simulink model "PlanarRobot5link_changedconstraint"  (R2022b)
settings: Solver=VariableStepAuto  StartTime=0.0  StopTime=100  RelTol=1e-3
values from neighbouring files (symbols this model uses):
  I = [1; 1; 1; 0.5; 0.5]*0.2    [RobDyn4link.m]
  l = [1; 1; 1; 1; 2]*0.2    [RobDyn4link.m]
  lc = l./2    [RobDyn4link.m]
  m = [1; 1; 1; 0.3; 0.3]*1    [RobDyn4link.m]
  q0 = [pi/2; -pi/4; -1*pi/6;-pi/12;0;]    [RobDyn4link.m]
  theta_max = [0.915*pi; 0.915*pi; 0.915*pi; 0.915*pi; 0.915*pi;]    [RobDyn4link.m]
  theta_min = [-0.915*pi; -0.915*pi; -0.915*pi; -0.915*pi; -0.915*pi;]    [RobDyn4link.m]
libraries: slpidlib x2
(part 1 of 3)
settings Model: Creator=yu  LastModifiedBy=ge89moy

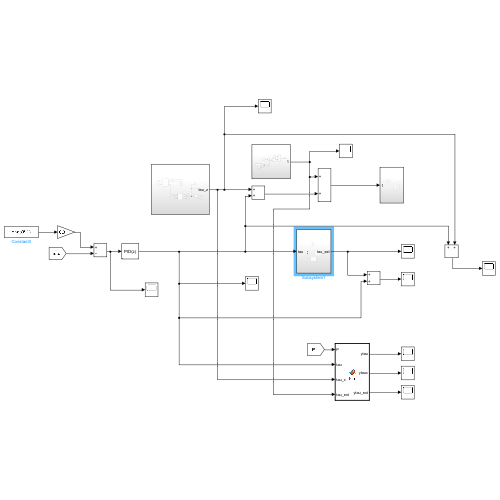
[thumbnail: Simulink's stored preview of the top-level diagram]
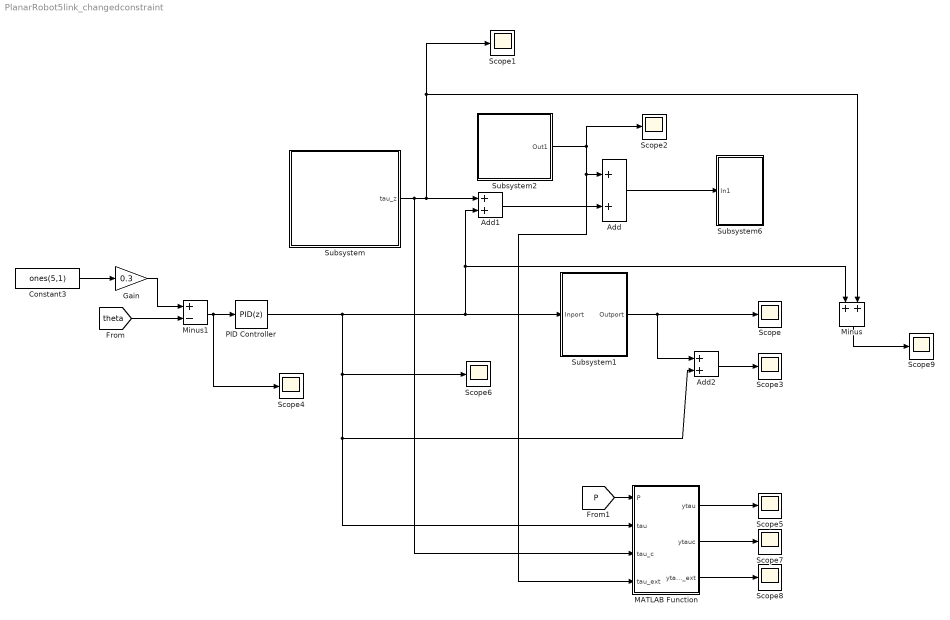
== system PlanarRobot5link_changedconstraint ==
  Add : Sum
  Add1 : Sum
  Add2 : Sum
  Constant3 : Constant  Value=ones(5,1)
  Gain : Gain  Gain=0.3
  MATLAB Function : MATLAB Function  TreatAsAtomicUnit=on
  Minus : Sum
  Minus1 : Sum  Inputs=+-
  PID Controller : slpidlib/PID Controller  Controller=PID  Form=Parallel  TimeDomain=Discrete-time  UseExternalTs=off  SampleTime=1e-3  IntegratorMethod=Forward Euler  FilterMethod=Forward Euler  ControllerParametersSource=internal  P=100  I=0  UseKiTs=off  D=50  N=100  UseFilter=on  TunerSelectOption=Transfer Function Based (PID Tuner App)  InitialConditionSource=internal  InitialConditionForIntegrator=0  InitialConditionForFilter=0  DifferentiatorICPrevScaledInput=0  ExternalReset=none  TrackingMode=off  Kt=1  LimitOutput=off  SatLimitsSource=internal  UpperSaturationLimit=inf  LowerSaturationLimit=-inf  LinearizeAsGain=on  AntiWindupMode=none  Kb=1  LimitIntegrator=off  UpperIntegratorSaturationLimit=inf  LowerIntegratorSaturationLimit=-inf  POutMin=[]  POutMax=[]  IOutMin=[]  IOutMax=[]  DOutMin=[]  DOutMax=[]  NOutMin=[]  NOutMax=[]  SumOutMin=[]  SumOutMax=[]  SaturationOutMin=[]  SaturationOutMax=[]  PParamMin=[]  PParamMax=[]  IParamMin=[]  IParamMax=[]  DParamMin=[]  DParamMax=[]  NParamMin=[]  NParamMax=[]  KbParamMin=[]  KbParamMax=[]  KtParamMin=[]  KtParamMax=[]  KbOutMin=[]  KbOutMax=[]  KtOutMin=[]  KtOutMax=[]  IntegratorOutMin=[]  IntegratorOutMax=[]  FilterOutMin=[]  FilterOutMax=[]  SumI1OutMin=[]  SumI1OutMax=[]  SumI2OutMin=[]  SumI2OutMax=[]  SumI3OutMin=[]  SumI3OutMax=[]  SumI4OutMin=[]  SumI4OutMax=[]  SumDOutMin=[]  SumDOutMax=[]  DifferentiatorOutMin=[]  DifferentiatorOutMax=[]  FilterDiffOutCoefMin=[]  FilterDiffOutCoefMax=[]  ReciprocalOutMin=[]  ReciprocalOutMax=[]  SumDenOutMin=[]  SumDenOutMax=[]  SumNumOutMin=[]  SumNumOutMax=[]  DivideOutMin=[]  DivideOutMax=[]  UdiffTsProdOutMin=[]  UdiffTsProdOutMax=[]  NTsProdOutMin=[]  NTsProdOutMax=[]  UintegralTsProdOutMin=[]  UintegralTsProdOutMax=[]  UngainTsProdOutMin=[]  UngainTsProdOutMax=[]  ClampingZeroOutDataTypeStr=Inherit: Inherit via back propagation  ClampingZeroOutMin=[]  ClampingZeroOutMax=[]  FilterDenConstantOutDataTypeStr=Inherit: Inherit via back propagation  FilterDenConstantOutMin=[]  FilterDenConstantOutMax=[]  PCopyOutDataTypeStr=Inherit: Inherit via back propagation  PCopyOutMin=[]  PCopyOutMax=[]  NCopyOutDataTypeStr=Inherit: Inherit via back propagation  NCopyOutMin=[]  NCopyOutMax=[]  IntegratorContinuousStateAttributes=''  IntegratorStateMustResolveToSignalObject=off  IntegratorRTWStateStorageClass=Auto  FilterContinuousStateAttributes=''  FilterStateMustResolveToSignalObject=off  FilterRTWStateStorageClass=Auto  ParallelPVariant=InternalParameters  IdealPVariant=Disabled  IVariant=InternalParameters  DVariant=InternalParameters  IntegratorVariant=Discrete  SatVariant=Disabled  AWVariant=Passthrough  PCopyVariant=Disabled  TRVariant=Disabled  FdbkBlocksVariant=Forward  IdealPFdbkVariant=Disabled  SatFdbkVariant=Disabled  DerivativeFilterVariant=ForwardEulerFilter  NVariant=InternalParameters  NCopyVariant=Disabled  FilterICVariant=InternalICsFilter  IntegratorICVariant=InternalICs  ExternalResetVariant=Disabled  TRSumVariant=Passthrough  SumFdbkVariant=Disabled  SumVariant=Sum_PID  TsampFilterVariant=InternalTs  TsampNgainVariant=Passthrough  TsampIntegralVariant=Passthrough  ExternalSaturationOutDataTypeStr=Inherit: Same as second input
  Scope{,1..9} (10 alike) : Scope
  Subsystem : Subsystem
  Subsystem1 : Subsystem
  Subsystem2 : Subsystem
  Subsystem6 : Subsystem
  wires:
  Minus1/1 -> Scope4/1, PID Controller/1
  Add1/1 -> Add/2
  Constant3/1 -> Gain/1
  [theta] -> Minus1/2
  Add/1 -> Subsystem6/1(In1)
  Gain/1 -> Minus1/1
  Subsystem/1(tau_z) -> Add1/1, Scope1/1, Minus/2, MATLAB Function/3(tau_c)
  PID Controller/1 -> Add1/2, Minus/1, Subsystem1/1(Inport), Add2/2, MATLAB Function/2(tau), Scope6/1
  Subsystem1/1(Outport) -> Add2/1, Scope/1
  Add2/1 -> Scope3/1
  [P] -> MATLAB Function/1(P)
  MATLAB Function/1(ytau) -> Scope5/1
  MATLAB Function/2(ytauc) -> Scope7/1
  MATLAB Function/3(ytau_ext) -> Scope8/1
  Subsystem2/1(Out1) -> Add/1, MATLAB Function/4(tau_ext), Scope2/1
  Minus/1 -> Scope9/1

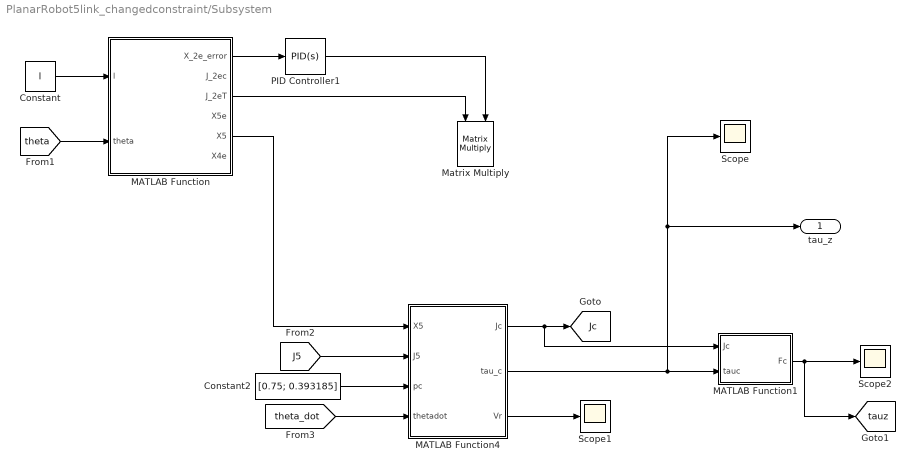
== system PlanarRobot5link_changedconstraint/Subsystem ==
  Constant : Constant  Value=l
  Constant2 : Constant  Value=[0.75; 0.393185]
  MATLAB Function : MATLAB Function  TreatAsAtomicUnit=on
  MATLAB Function1 : MATLAB Function  TreatAsAtomicUnit=on
  MATLAB Function4 : MATLAB Function  TreatAsAtomicUnit=on
  Matrix Multiply : Product  Multiplication=Matrix(*)
  PID Controller1 : slpidlib/PID Controller  Controller=PID  Form=Parallel  TimeDomain=Continuous-time  UseExternalTs=off  SampleTime=-1  IntegratorMethod=Forward Euler  FilterMethod=Forward Euler  ControllerParametersSource=internal  P=1e5  I=0  UseKiTs=off  D=1e3  N=100  UseFilter=on  TunerSelectOption=Transfer Function Based (PID Tuner App)  InitialConditionSource=internal  InitialConditionForIntegrator=0  InitialConditionForFilter=0  DifferentiatorICPrevScaledInput=0  ExternalReset=none  TrackingMode=off  Kt=1  LimitOutput=off  SatLimitsSource=internal  UpperSaturationLimit=inf  LowerSaturationLimit=-inf  LinearizeAsGain=on  AntiWindupMode=none  Kb=1  LimitIntegrator=off  UpperIntegratorSaturationLimit=inf  LowerIntegratorSaturationLimit=-inf  POutMin=[]  POutMax=[]  IOutMin=[]  IOutMax=[]  DOutMin=[]  DOutMax=[]  NOutMin=[]  NOutMax=[]  SumOutMin=[]  SumOutMax=[]  SaturationOutMin=[]  SaturationOutMax=[]  PParamMin=[]  PParamMax=[]  IParamMin=[]  IParamMax=[]  DParamMin=[]  DParamMax=[]  NParamMin=[]  NParamMax=[]  KbParamMin=[]  KbParamMax=[]  KtParamMin=[]  KtParamMax=[]  KbOutMin=[]  KbOutMax=[]  KtOutMin=[]  KtOutMax=[]  IntegratorOutMin=[]  IntegratorOutMax=[]  FilterOutMin=[]  FilterOutMax=[]  SumI1OutMin=[]  SumI1OutMax=[]  SumI2OutMin=[]  SumI2OutMax=[]  SumI3OutMin=[]  SumI3OutMax=[]  SumI4OutMin=[]  SumI4OutMax=[]  SumDOutMin=[]  SumDOutMax=[]  DifferentiatorOutMin=[]  DifferentiatorOutMax=[]  FilterDiffOutCoefMin=[]  FilterDiffOutCoefMax=[]  ReciprocalOutMin=[]  ReciprocalOutMax=[]  SumDenOutMin=[]  SumDenOutMax=[]  SumNumOutMin=[]  SumNumOutMax=[]  DivideOutMin=[]  DivideOutMax=[]  UdiffTsProdOutMin=[]  UdiffTsProdOutMax=[]  NTsProdOutMin=[]  NTsProdOutMax=[]  UintegralTsProdOutMin=[]  UintegralTsProdOutMax=[]  UngainTsProdOutMin=[]  UngainTsProdOutMax=[]  ClampingZeroOutDataTypeStr=Inherit: Inherit via back propagation  ClampingZeroOutMin=[]  ClampingZeroOutMax=[]  FilterDenConstantOutDataTypeStr=Inherit: Inherit via back propagation  FilterDenConstantOutMin=[]  FilterDenConstantOutMax=[]  PCopyOutDataTypeStr=Inherit: Inherit via back propagation  PCopyOutMin=[]  PCopyOutMax=[]  NCopyOutDataTypeStr=Inherit: Inherit via back propagation  NCopyOutMin=[]  NCopyOutMax=[]  IntegratorContinuousStateAttributes=''  IntegratorStateMustResolveToSignalObject=off  IntegratorRTWStateStorageClass=Auto  FilterContinuousStateAttributes=''  FilterStateMustResolveToSignalObject=off  FilterRTWStateStorageClass=Auto  ParallelPVariant=InternalParameters  IdealPVariant=Disabled  IVariant=InternalParameters  DVariant=InternalParameters  IntegratorVariant=Continuous  SatVariant=Disabled  AWVariant=Passthrough  PCopyVariant=Disabled  TRVariant=Disabled  FdbkBlocksVariant=Forward  IdealPFdbkVariant=Disabled  SatFdbkVariant=Disabled  DerivativeFilterVariant=ContFilter  NVariant=InternalParameters  NCopyVariant=Disabled  FilterICVariant=InternalICsFilter  IntegratorICVariant=InternalICs  ExternalResetVariant=Disabled  TRSumVariant=Passthrough  SumFdbkVariant=Disabled  SumVariant=Sum_PID  TsampFilterVariant=InternalTs  TsampNgainVariant=Passthrough  TsampIntegralVariant=Passthrough  ExternalSaturationOutDataTypeStr=Inherit: Same as second input
  Scope : Scope
  Scope1 : Scope
  Scope2 : Scope
  tau_z : Outport
  tag scope: Jc=global, tauz=global
  wires:
  MATLAB Function4/2(tau_c) -> MATLAB Function1/2(tauc), Scope/1, tau_z/1
  PID Controller1/1 -> Matrix Multiply/2
  Constant/1 -> MATLAB Function/1(l)
  [theta] -> MATLAB Function/2(theta)
  MATLAB Function/3(J_2eT) -> Matrix Multiply/1
  MATLAB Function/1(X_2e_error) -> PID Controller1/1
  MATLAB Function/5(X5) -> MATLAB Function4/1(X5)
  Constant2/1 -> MATLAB Function4/3(pc)
  [J5] -> MATLAB Function4/2(J5)
  [theta_dot] -> MATLAB Function4/4(thetadot)
  MATLAB Function4/1(Jc) -> MATLAB Function1/1(Jc), [Jc]
  MATLAB Function4/3(Vr) -> Scope1/1
  MATLAB Function1/1(Fc) -> [tauz], Scope2/1

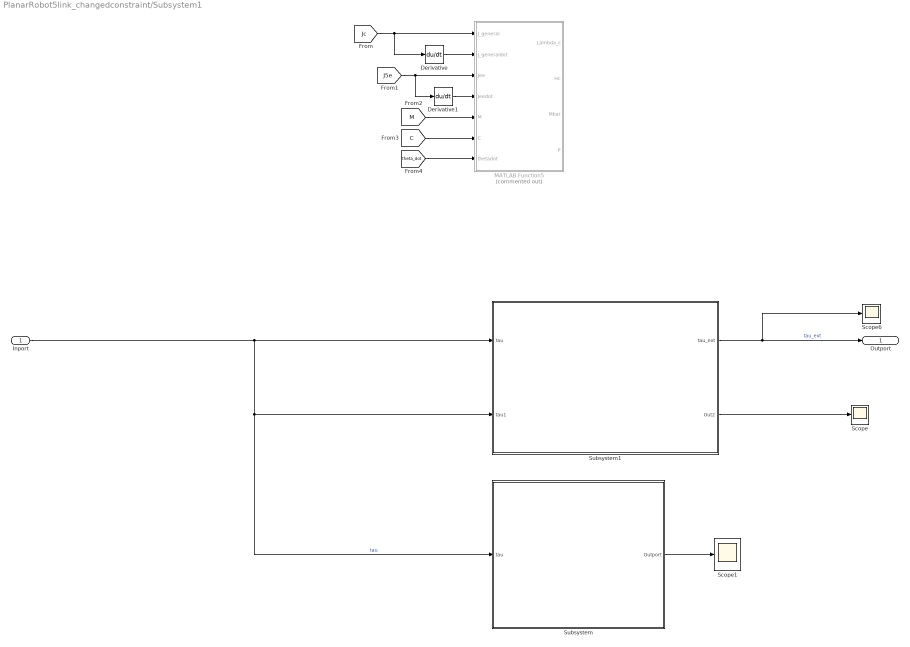
== system PlanarRobot5link_changedconstraint/Subsystem1 ==
  Inport : Inport
  Derivative : Derivative
  Derivative1 : Derivative
  MATLAB Function5 : MATLAB Function  Commented=on  TreatAsAtomicUnit=on
  Scope : Scope
  Scope1 : Scope
  Scope6 : Scope
  Subsystem : Subsystem
  Subsystem1 : Subsystem
  Outport : Outport
  wires:
  Inport/1 -> Subsystem/1(tau), Subsystem1/2(tau1), Subsystem1/1(tau)  "tau"
  Subsystem/1(Outport) -> Scope1/1
  Subsystem1/1(tau_ext) -> Outport/1, Scope6/1  "tau_ext"
  Subsystem1/2(Out2) -> Scope/1
  [Jc] -> Derivative/1, MATLAB Function5/1(J_general)
  Derivative/1 -> MATLAB Function5/2(J_generaldot)
  [J5e] -> Derivative1/1, MATLAB Function5/3(Jee)
  Derivative1/1 -> MATLAB Function5/4(Jeedot)
  [M] -> MATLAB Function5/5(M)
  [C] -> MATLAB Function5/6(C)
  [theta_dot] -> MATLAB Function5/7(thetadot)

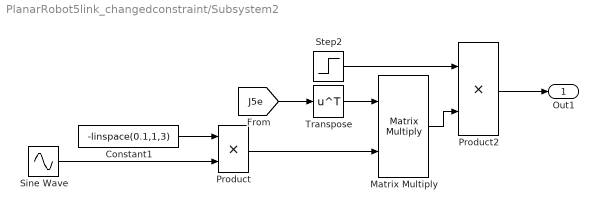
== system PlanarRobot5link_changedconstraint/Subsystem2 ==
  Constant1 : Constant  Value=-linspace(0.1,1,3)
  Matrix Multiply : Product  Multiplication=Matrix(*)
  Product : Product
  Product2 : Product
  Sine Wave : Sin  Frequency=0.1  SampleTime=0
  Step2 : Step  Time=15  After=5  SampleTime=0
  Transpose : Math  Operator=transpose
  Out1 : Outport
  wires:
  [J5e] -> Transpose/1
  Transpose/1 -> Matrix Multiply/1
  Product/1 -> Matrix Multiply/2
  Matrix Multiply/1 -> Product2/2
  Product2/1 -> Out1/1
  Step2/1 -> Product2/1
  Constant1/1 -> Product/1
  Sine Wave/1 -> Product/2

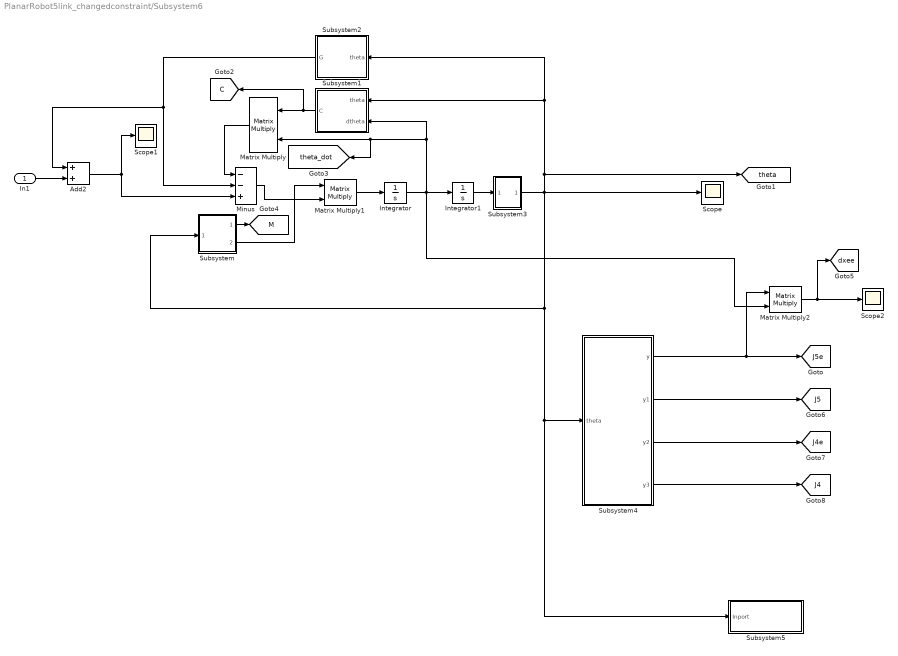
== system PlanarRobot5link_changedconstraint/Subsystem6 ==
  In1 : Inport
  Add2 : Sum
  Integrator : Integrator
  Integrator1 : Integrator  InitialCondition=q0
  Matrix Multiply : Product  Multiplication=Matrix(*)
  Matrix Multiply1 : Product  Multiplication=Matrix(*)
  Matrix Multiply2 : Product  Multiplication=Matrix(*)
  Minus : Sum  Inputs=--+
  Scope : Scope
  Scope1 : Scope
  Scope2 : Scope
  Subsystem : Subsystem
  Subsystem1 : Subsystem
  Subsystem2 : Subsystem
  Subsystem3 : Subsystem
  Subsystem4 : Subsystem
  Subsystem5 : Subsystem
  tag scope: C=global, J4=global, J4e=global, J5=global, J5e=global, M=global, dxee=global, theta=global, theta_dot=global
  wires:
  Subsystem2/1(G) -> Add2/1, Minus/2
  Subsystem/2(Outport1) -> Matrix Multiply1/1
  Subsystem/1(Outport) -> [M]
  In1/1 -> Add2/2
  Integrator1/1 -> Subsystem3/1(In1)
  Integrator/1 -> Matrix Multiply2/2, Integrator1/1, Subsystem1/2(dtheta), Matrix Multiply/2, [theta_dot]
  Subsystem4/2(y1) -> [J5]
  Subsystem4/4(y3) -> [J4]
  Matrix Multiply/1 -> Minus/1
  Add2/1 -> Scope1/1, Minus/3
  Subsystem4/3(y2) -> [J4e]
  Subsystem3/1(theta) -> Subsystem4/1(theta), Subsystem5/1(Inport), Subsystem/1(Inport), Subsystem1/1(theta), Subsystem2/1(theta), [theta], Scope/1
  Matrix Multiply1/1 -> Integrator/1
  Subsystem4/1(y) -> [J5e], Matrix Multiply2/1
  Subsystem1/1(C) -> [C], Matrix Multiply/1
  Minus/1 -> Matrix Multiply1/2
  Matrix Multiply2/1 -> Scope2/1, [dxee]

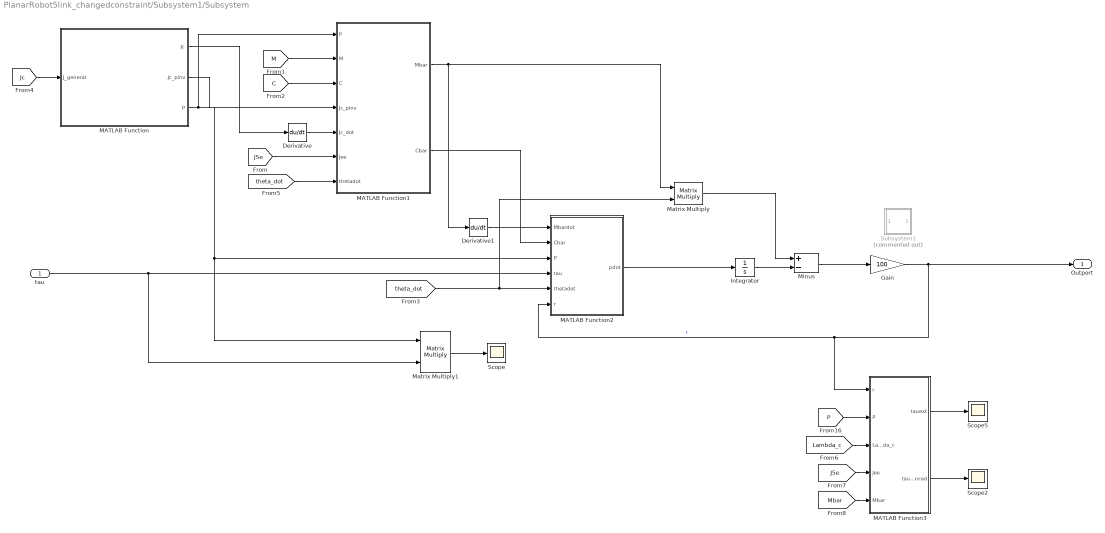
== system PlanarRobot5link_changedconstraint/Subsystem1/Subsystem ==
  tau : Inport
  Derivative : Derivative
  Derivative1 : Derivative
  Gain : Gain  Gain=100
  Integrator : Integrator
  MATLAB Function : MATLAB Function  TreatAsAtomicUnit=on
  MATLAB Function1 : MATLAB Function  TreatAsAtomicUnit=on
  MATLAB Function2 : MATLAB Function  TreatAsAtomicUnit=on
  MATLAB Function3 : MATLAB Function  TreatAsAtomicUnit=on
  Matrix Multiply : Product  Multiplication=Matrix(*)
  Matrix Multiply1 : Product  Multiplication=Matrix(*)
  Minus : Sum  Inputs=+-
  Scope : Scope
  Scope2 : Scope
  Scope5 : Scope
  Subsystem1 : Subsystem  Commented=on
  Outport : Outport
  wires:
  [Jc] -> MATLAB Function/1(J_general)
  MATLAB Function/2(Jc_pinv) -> MATLAB Function1/4(Jc_pinv)
  MATLAB Function1/1(Mbar) -> Derivative1/1, Matrix Multiply/1
  MATLAB Function/1(Jc) -> Derivative/1
  Derivative/1 -> MATLAB Function1/5(Jc_dot)
  [M] -> MATLAB Function1/2(M)
  [C] -> MATLAB Function1/3(C)
  tau/1 -> Matrix Multiply1/2, MATLAB Function2/4(tau)
  [theta_dot] -> Matrix Multiply/2, MATLAB Function2/5(thetadot)
  MATLAB Function2/1(pdot) -> Integrator/1
  Matrix Multiply/1 -> Minus/1
  Integrator/1 -> Minus/2
  Minus/1 -> Gain/1
  MATLAB Function/3(P) -> Matrix Multiply1/1, MATLAB Function2/3(P), MATLAB Function1/1(P)
  Matrix Multiply1/1 -> Scope/1
  MATLAB Function1/2(Cbar) -> MATLAB Function2/2(Cbar)
  Gain/1 -> MATLAB Function2/6(r), MATLAB Function3/1(r), Outport/1  "r"
  [J5e] -> MATLAB Function1/6(Jee)
  [theta_dot] -> MATLAB Function1/7(thetadot)
  Derivative1/1 -> MATLAB Function2/1(Mbardot)
  [Lambda_c] -> MATLAB Function3/3(Lambda_c)
  [Mbar] -> MATLAB Function3/5(Mbar)
  [J5e] -> MATLAB Function3/4(Jee)
  [P] -> MATLAB Function3/2(P)
  MATLAB Function3/1(tauext) -> Scope5/1
  MATLAB Function3/2(tau_ext_enhanced) -> Scope2/1

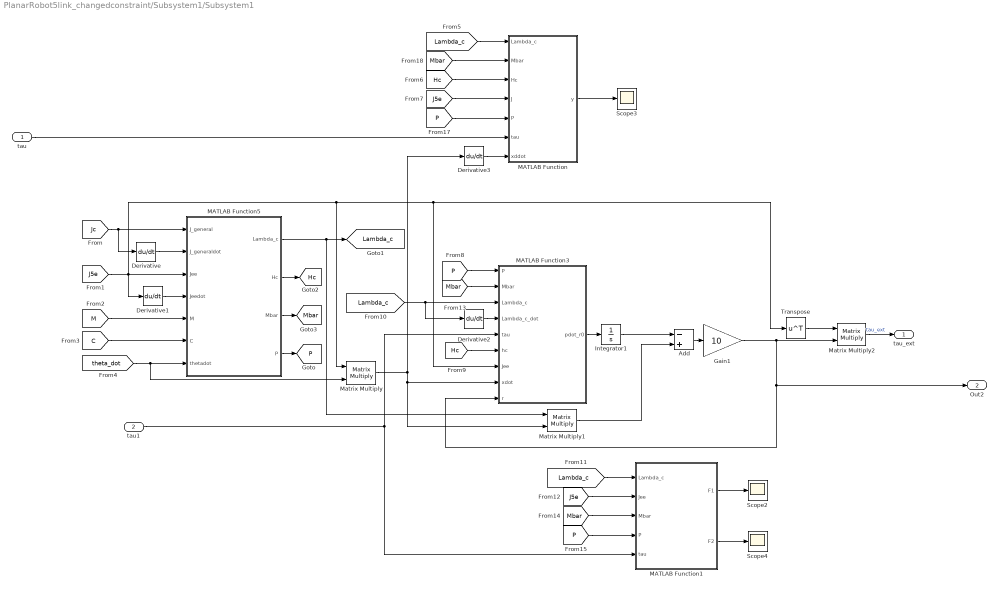
== system PlanarRobot5link_changedconstraint/Subsystem1/Subsystem1 ==
  tau : Inport
  tau1 : Inport  Port=2
  Add : Sum  Inputs=-+
  Derivative{,1..3} (4 alike) : Derivative
  Gain1 : Gain  Gain=10
  Integrator1 : Integrator
  MATLAB Function : MATLAB Function  TreatAsAtomicUnit=on
  MATLAB Function1 : MATLAB Function  TreatAsAtomicUnit=on
  MATLAB Function3 : MATLAB Function  TreatAsAtomicUnit=on
  MATLAB Function5 : MATLAB Function  TreatAsAtomicUnit=on
  Matrix Multiply : Product  Multiplication=Matrix(*)
  Matrix Multiply1 : Product  Multiplication=Matrix(*)
  Matrix Multiply2 : Product  Multiplication=Matrix(*)
  Scope2 : Scope
  Scope3 : Scope
  Scope4 : Scope
  Transpose : Math  Operator=transpose
  tau_ext : Outport
  Out2 : Outport  Port=2
  tag scope: Hc=global, Lambda_c=global, Mbar=global, P=global
  wires:
  Matrix Multiply1/1 -> Add/2
  [Mbar] -> MATLAB Function3/2(Mbar)
  [M] -> MATLAB Function5/5(M)
  [Lambda_c] -> MATLAB Function/1(Lambda_c)
  Transpose/1 -> Matrix Multiply2/1
  Derivative/1 -> MATLAB Function5/2(J_generaldot)
  Add/1 -> Gain1/1
  [C] -> MATLAB Function5/6(C)
  [J5e] -> MATLAB Function1/2(Jee)
  [Mbar] -> MATLAB Function/2(Mbar)
  [Lambda_c] -> Derivative2/1, MATLAB Function3/3(Lambda_c)
  tau/1 -> MATLAB Function/6(tau)
  MATLAB Function1/2(F2) -> Scope4/1
  MATLAB Function5/4(P) -> [P]
  [theta_dot] -> Matrix Multiply/2, MATLAB Function5/7(thetadot)
  [P] -> MATLAB Function1/4(P)
  Derivative2/1 -> MATLAB Function3/4(Lambda_c_dot)
  MATLAB Function3/1(pdot_r0) -> Integrator1/1
  [Hc] -> MATLAB Function/3(Hc)
  MATLAB Function5/1(Lambda_c) -> [Lambda_c], Matrix Multiply1/1
  Derivative1/1 -> MATLAB Function5/4(Jeedot)
  Derivative3/1 -> MATLAB Function/7(xddot)
  Matrix Multiply/1 -> Derivative3/1, MATLAB Function3/8(xdot), Matrix Multiply1/2
  [P] -> MATLAB Function3/1(P)
  MATLAB Function/1(y) -> Scope3/1
  Matrix Multiply2/1 -> tau_ext/1  "tau_ext"
  [J5e] -> MATLAB Function/4(J)
  MATLAB Function1/1(F1) -> Scope2/1
  [Lambda_c] -> MATLAB Function1/1(Lambda_c)
  [Hc] -> MATLAB Function3/6(hc)
  [P] -> MATLAB Function/5(P)
  [J5e] -> MATLAB Function3/7(Jee), Transpose/1, Matrix Multiply/1, MATLAB Function5/3(Jee), Derivative1/1
  [Jc] -> Derivative/1, MATLAB Function5/1(J_general)
  [Mbar] -> MATLAB Function1/3(Mbar)
  tau1/1 -> MATLAB Function1/5(tau), MATLAB Function3/5(tau)
  MATLAB Function5/2(Hc) -> [Hc]
  MATLAB Function5/3(Mbar) -> [Mbar]
  Gain1/1 -> Matrix Multiply2/2, Out2/1, MATLAB Function3/9(r)
  Integrator1/1 -> Add/1

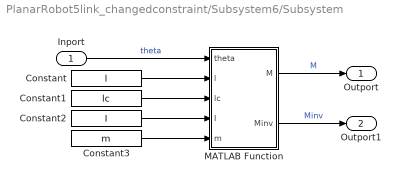
== system PlanarRobot5link_changedconstraint/Subsystem6/Subsystem ==
  Inport : Inport  PortDimensions=[5,1]
  Constant : Constant  Value=l
  Constant1 : Constant  Value=lc
  Constant2 : Constant  Value=I
  Constant3 : Constant  Value=m
  MATLAB Function : MATLAB Function  TreatAsAtomicUnit=on
  Outport : Outport  PortDimensions=[5,5]
  Outport1 : Outport  Port=2  PortDimensions=[5,5]
  wires:
  Constant3/1 -> MATLAB Function/5(m)
  MATLAB Function/1(M) -> Outport/1  "M"
  Inport/1 -> MATLAB Function/1(theta)  "theta"
  Constant2/1 -> MATLAB Function/4(I)
  Constant/1 -> MATLAB Function/2(l)
  Constant1/1 -> MATLAB Function/3(lc)
  MATLAB Function/2(Minv) -> Outport1/1  "Minv"

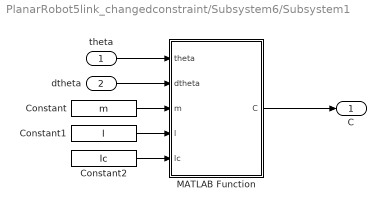
== system PlanarRobot5link_changedconstraint/Subsystem6/Subsystem1 ==
  theta : Inport  PortDimensions=[5,1]
  dtheta : Inport  Port=2  PortDimensions=[5,1]
  Constant : Constant  Value=m
  Constant1 : Constant  Value=l
  Constant2 : Constant  Value=lc
  MATLAB Function : MATLAB Function  TreatAsAtomicUnit=on
  C : Outport  PortDimensions=[5,5]
  wires:
  theta/1 -> MATLAB Function/1(theta)
  MATLAB Function/1(C) -> C/1
  dtheta/1 -> MATLAB Function/2(dtheta)
  Constant/1 -> MATLAB Function/3(m)
  Constant2/1 -> MATLAB Function/5(lc)
  Constant1/1 -> MATLAB Function/4(l)

== system PlanarRobot5link_changedconstraint/Subsystem6/Subsystem2 ==
  theta : Inport  PortDimensions=[5,1]
  Constant : Constant  Value=m
  Constant1 : Constant  Value=l
  Constant2 : Constant  Value=lc
  MATLAB Function : MATLAB Function  TreatAsAtomicUnit=on
  G : Outport  PortDimensions=[5,1]
  wires:
  Constant1/1 -> MATLAB Function/3(l)
  Constant2/1 -> MATLAB Function/4(lc)
  Constant/1 -> MATLAB Function/2(m)
  MATLAB Function/1(G) -> G/1
  theta/1 -> MATLAB Function/1(theta)

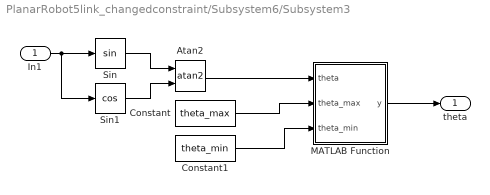
== system PlanarRobot5link_changedconstraint/Subsystem6/Subsystem3 ==
  In1 : Inport
  Atan2 : Trigonometry  Operator=atan2
  Constant : Constant  Value=theta_max
  Constant1 : Constant  Value=theta_min
  MATLAB Function : MATLAB Function  TreatAsAtomicUnit=on
  Sin : Trigonometry
  Sin1 : Trigonometry  Operator=cos
  theta : Outport  PortDimensions=[5,1]
  wires:
  Atan2/1 -> MATLAB Function/1(theta)
  In1/1 -> Sin1/1, Sin/1
  Sin/1 -> Atan2/1
  Sin1/1 -> Atan2/2
  MATLAB Function/1(y) -> theta/1
  Constant/1 -> MATLAB Function/2(theta_max)
  Constant1/1 -> MATLAB Function/3(theta_min)

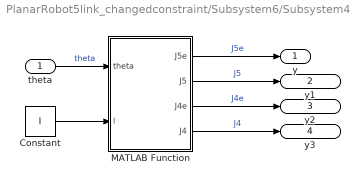
== system PlanarRobot5link_changedconstraint/Subsystem6/Subsystem4 ==
  theta : Inport
  Constant : Constant  Value=l
  MATLAB Function : MATLAB Function  TreatAsAtomicUnit=on
  y : Outport
  y1 : Outport  Port=2
  y2 : Outport  Port=3
  y3 : Outport  Port=4
  wires:
  theta/1 -> MATLAB Function/1(theta)  "theta"
  MATLAB Function/1(J5e) -> y/1  "J5e"
  Constant/1 -> MATLAB Function/2(l)
  MATLAB Function/2(J5) -> y1/1  "J5"
  MATLAB Function/3(J4e) -> y2/1  "J4e"
  MATLAB Function/4(J4) -> y3/1  "J4"

== system PlanarRobot5link_changedconstraint/Subsystem6/Subsystem5 ==
  Inport : Inport
  Constant : Constant  Value=l
  MATLAB Function : MATLAB Function  Commented=on  TreatAsAtomicUnit=on
  MATLAB Function1 : MATLAB Function  TreatAsAtomicUnit=on
  To Workspace : ToWorkspace  VariableName=Xlink  SaveFormat=Timeseries  SampleTime=-1
  To Workspace1 : ToWorkspace  VariableName=Ylink  SaveFormat=Timeseries  SampleTime=-1
  wires:
  MATLAB Function1/1(x) -> To Workspace/1, MATLAB Function/1(x)
  MATLAB Function1/2(y) -> To Workspace1/1, MATLAB Function/2(y)
  Inport/1 -> MATLAB Function1/1(theta)  "theta"
  Constant/1 -> MATLAB Function1/2(l)

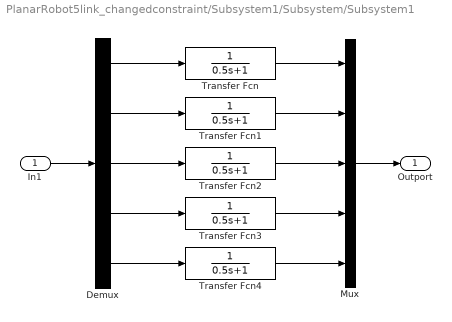
== system PlanarRobot5link_changedconstraint/Subsystem1/Subsystem/Subsystem1 ==
  In1 : Inport
  Demux : Demux  Outputs=5
  Mux : Mux  Inputs=5
  Transfer Fcn{,1..4} (5 alike) : TransferFcn  Denominator=[0.5 1]
  Outport : Outport
  wires:
  Mux/1 -> Outport/1
  Transfer Fcn4/1 -> Mux/5
  Transfer Fcn3/1 -> Mux/4
  Transfer Fcn2/1 -> Mux/3
  Transfer Fcn1/1 -> Mux/2
  Transfer Fcn/1 -> Mux/1
  Demux/2 -> Transfer Fcn1/1
  Demux/3 -> Transfer Fcn2/1
  Demux/4 -> Transfer Fcn3/1
  Demux/1 -> Transfer Fcn/1
  In1/1 -> Demux/1
  Demux/5 -> Transfer Fcn4/1

== matlab function PlanarRobot5link_changedconstraint/MATLAB Function ==
  data: P input; ytau output; tau input; tau_c input; tau_ext input; ytauc output; ytau_ext output
function [ytau,ytauc,ytau_ext]= fcn(P,tau,tau_c,tau_ext)

ytau = P*tau;
ytauc = P*tau_c;
ytau_ext = P*tau_ext;

== matlab function PlanarRobot5link_changedconstraint/Subsystem1/Subsystem1/MATLAB Function1 ==
  data: Lambda_c input; F1 output; Jee input; Mbar input; P input; tau input; F2 output
function [F1,F2]= fcn(Lambda_c,Jee,Mbar,P,tau)

F1 = Lambda_c*Jee/Mbar*P*tau;
F2 = (Jee'/(Jee*Jee'))'*tau;

== matlab function PlanarRobot5link_changedconstraint/Subsystem1/Subsystem1/MATLAB Function ==
  data: Lambda_c input; Mbar input; y output; Hc input; J input; P input; tau input; xddot input
function y = fcn(Lambda_c, Mbar, Hc, J,P,tau, xddot)
% J_pinv = J'/(J*J');
% y =J'*(J_pinv'*tau - Lambda_c*xddot - Hc);

y = -J'*Lambda_c*J/Mbar*P*tau + J'*Lambda_c*xddot + J'*Hc;

== matlab function PlanarRobot5link_changedconstraint/Subsystem/MATLAB Function1 ==
  data: Jc input; tauc input; Fc output
function Fc = fcn(Jc, tauc)
Fc = (Jc'/(Jc*Jc'))'*tauc;

% y = u;

== matlab function PlanarRobot5link_changedconstraint/Subsystem1/Subsystem/MATLAB Function3 ==
  data: r input; tauext output; P input; Lambda_c input; Jee input; Mbar input; tau_ext_enhanced output
function [tauext,tau_ext_enhanced]= fcn(r, P,Lambda_c,Jee,Mbar)

tauext = P'/(P*P' + 1e-3*eye(5))*r;
tau_ext_enhanced = Jee'*Lambda_c*Jee/Mbar*P*r;

== matlab function PlanarRobot5link_changedconstraint/Subsystem1/MATLAB Function5 ==
  data: Lambda_c output size=[3,3]; Hc output; J_general input; J_generaldot input; Jee input; Jeedot input; M input; C input; thetadot input; Mbar output; P output
function [Lambda_c,Hc,Mbar,P] = fcn(J_general,J_generaldot,Jee,Jeedot,M,C,thetadot)
Jc = J_general;
Jc_pinv = Jc'/(Jc*Jc' + 0*eye(1));
P = eye(5) - Jc_pinv*Jc;

%% previous part
Pnull = eye(5) - P;
Mc = P*M + (eye(5) - P);
Lambda_c = (Jee * (Mc \ P) * Jee'+ 1e-3*eye(3) ) \ eye(3);
% 
% PMP = P*M*P;
% McInvP = PMP'*(PMP*PMP');
% % Lambda_c = eye(3)/(Jee*McInvP*Jee'+1e-1*eye(3));
% 
% coder.extrinsic('computeLambdaC');
% Lambda_c = eye(3);
% Lambda_c = computeLambdaC(Jee,Mc,P,1e-6);

%% Farhad Aghili 2016 ICRA
% nv = 0.5;
% Mbar = P*M*P + nv*(eye(5) - P);
% S = eye(5) - M/Mbar*P;
% Jcdot = J_generaldot;
% Gamma = -Jc_pinv*Jcdot;
% Omega = Gamma - Gamma';
% 
% Lambda_c = (Jee/Mbar*P*Jee');
% Hc = Lambda_c*(Jee/Mbar*(Mbar*S'*Omega*thetadot + P*C*thetadot) - Jeedot*thetadot);

== matlab function PlanarRobot5link_changedconstraint/Subsystem/MATLAB Function4 ==
  data: X5 input; J5 input; Jc output; pc input; tau_c output; thetadot input; Vr output
function [Jc,tau_c,Vr] = fcn(X5, J5, pc,thetadot)
pr = X5(1:2);
theta4 = X5(3);

R = [cos(theta4), -sin(theta4); sin(theta4), cos(theta4)];
y = R(:,2);
dir = pr - pc;
A = [-y(1), y(2), dir(2)*y(2) - dir(1)*y(1)];
Jc = A*J5;

Vr = Jc*thetadot;

prdot = J5*thetadot;
Fcol = 10*(pc(2) - pr(2)) - 5*prdot(2);

% size(Jc)
tau_z = Jc'*-10;
tau_c = [tau_z];

== matlab function PlanarRobot5link_changedconstraint/Subsystem1/Subsystem1/MATLAB Function3 ==
  data: P input; Mbar input; Lambda_c input; Lambda_c_dot input; pdot_r0 output; tau input; hc input; Jee input; xdot input; r input
function pdot_r0 = fcn(P,Mbar,Lambda_c,Lambda_c_dot,tau,hc,Jee,xdot,r)
% Jee_pinv = Jee'/(Jee*Jee' + 1e-3*eye(3));
F = Lambda_c*Jee/Mbar*P*tau;
% % F = Jee_pinv'*tau;
pdot_r0 = Lambda_c_dot*xdot + F - hc + r;

== matlab function PlanarRobot5link_changedconstraint/Subsystem1/Subsystem/MATLAB Function ==
  data: J_general input; Jc output; Jc_pinv output; P output
function [Jc, Jc_pinv, P] = fcn(J_general)
Jc = J_general;
Jc_pinv = Jc'/(Jc*Jc');
P = eye(5) - Jc_pinv*Jc;

== matlab function PlanarRobot5link_changedconstraint/Subsystem1/Subsystem/MATLAB Function1 ==
  data: P input; Mbar output; M input; C input; Jc_pinv input; Jc_dot input; Cbar output; Jee input; thetadot input
function [Mbar,Cbar] = fcn(P,M,C,Jc_pinv,Jc_dot,Jee,thetadot)
% Pdot = -Jc_pinv*Jc_dot*P - P*Jc_dot'*Jc_pinv';
% Mbar = P*M*P + eye(5) - P;
% Cbar = P*C*P + P*M*Pdot*P + Jc_pinv*Jc_dot*P;


nv = 0.5;
Mbar = P*M*P + nv*(eye(5) - P);
S = eye(5) - M/Mbar*P;
Gamma = -Jc_pinv*Jc_dot;
Omega = Gamma - Gamma';
% Mbar = (Jee*(Mbar \ P)*Jee');
% Hc = Lambda_c*(Jee/Mbar*(S'*Omega*thetadot + P*C*thetadot) - Jeedot*thetadot);
Cbar = Mbar*S'*Omega*thetadot + P*C*thetadot;

== matlab function PlanarRobot5link_changedconstraint/Subsystem1/Subsystem/MATLAB Function2 ==
  data: Mbardot input; Cbar input; pdot output; P input; tau input; thetadot input; r input
function pdot = fcn(Mbardot,Cbar,P,tau,thetadot,r)

pdot = Mbardot*thetadot + P*tau - Cbar + r;
